simulink model "Model"  (R2020a)
settings: Solver=FixedStepAuto  StartTime=0.0  StopTime=20  RelTol=1e-3
undefined symbols (not defined in the file): A, B, Bv, Bvn, Bw, C, Cv, Cvn, Cw, d, D, DiscIntNeverNeededParam, J, K_fsfb, K_int, Kt, l, M, r, Ti, Ts
libraries: simulink x1
settings Model: Creator=User  LastModifiedBy=User
settings SolverCC: ZeroCrossControl=EnableAll  ZeroCrossAlgorithm=Adaptive
settings DebuggingCC: IgnoredZcDiagnostic=none

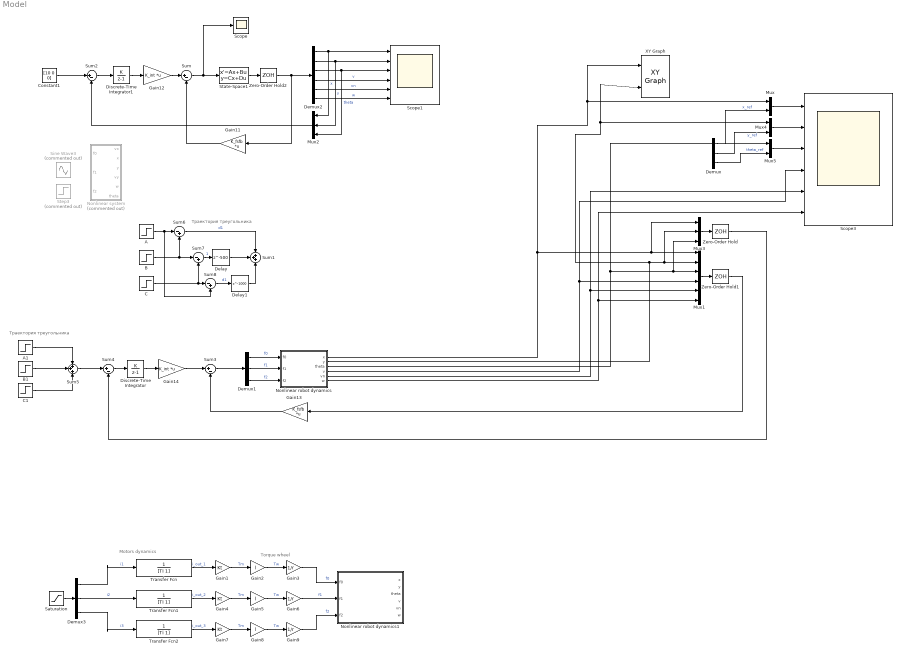
== system Model ==
  note: Motors dynamics
  note: Torque wheel
  note: Траектория треугольника
  note: Траектория треугольника
  A : Step  Time=0  Before=[0 0 0]  After=[0 0 0]  SampleTime=0
  A1 : Step  Time=0  Before=[0 0 0]  After=[0.5 -sqrt(3)/2 1]  SampleTime=0
  B : Step  Time=0  Before=[0.5 -sqrt(3)/2 0]  After=[0.5 -sqrt(3)/2 0]  SampleTime=Ts
  B1 : Step  Time=6  Before=[0 0 0]  After=[-1 0 1]  SampleTime=Ts
  C : Step  Time=0  Before=[-0.5 -sqrt(3)/2 0]  After=[-0.5 -sqrt(3)/2 0]  SampleTime=Ts
  C1 : Step  Time=12  Before=[0 0 0]  After=[0.5 sqrt(3)/2 0]  SampleTime=Ts
  Constant1 : Constant  Value=[10 0 0]
  Delay : Delay  DelayLength=500
  Delay1 : Delay  DelayLength=1000
  Demux : Demux  Outputs=3
  Demux1 : Demux  Outputs=3
  Demux2 : Demux  Outputs=6
  Demux3 : Demux  Outputs=3
  Discrete-Time Integrator : DiscreteIntegrator  IntegratorMethod=Accumulation: Forward Euler  SampleTime=Ts  ICPrevOutput=DiscIntNeverNeededParam  ICPrevScaledInput=DiscIntNeverNeededParam
  Discrete-Time Integrator1 : DiscreteIntegrator  IntegratorMethod=Accumulation: Forward Euler  SampleTime=Ts  ICPrevOutput=DiscIntNeverNeededParam  ICPrevScaledInput=DiscIntNeverNeededParam
  Gain1 : Gain  Gain=Kt
  Gain11 : Gain  Gain=K_fsfb  Multiplication=Matrix(K*u) (u vector)
  Gain12 : Gain  Gain=K_int  Multiplication=Matrix(K*u) (u vector)
  Gain13 : Gain  Gain=K_fsfb  Multiplication=Matrix(K*u) (u vector)
  Gain14 : Gain  Gain=K_int  Multiplication=Matrix(K*u) (u vector)
  Gain2 : Gain  Gain=l
  Gain3 : Gain  Gain=1/r
  Gain4 : Gain  Gain=Kt
  Gain5 : Gain  Gain=l
  Gain6 : Gain  Gain=1/r
  Gain7 : Gain  Gain=Kt
  Gain8 : Gain  Gain=l
  Gain9 : Gain  Gain=1/r
  Mux : Mux  Inputs=2
  Mux1 : Mux  Inputs=6
  Mux2 : Mux  Inputs=3
  Mux3 : Mux  Inputs=3
  Mux4 : Mux  Inputs=2
  Mux5 : Mux  Inputs=2
  Nonlinear robot dynamics : Subsystem
  Nonlinear robot dynamics1 : Subsystem
  Nonlinear system : Subsystem  Commented=on
  Saturation : Saturate  UpperLimit=4  LowerLimit=0
  Scope : Scope
  Scope1 : Scope  NumInputPorts=6
  Scope3 : Scope  NumInputPorts=6
  Sine Wave3 : Sin  Commented=on  SampleTime=0
  State-Space1 : StateSpace  A=A  B=B  C=C  D=D  InitialCondition=0  AbsoluteTolerance=-1
  Step3 : Step  Commented=on  Time=0  After=-5  SampleTime=0
  Sum{,2..4} (4 alike) : Sum  Inputs=|+-
  Sum1 : Sum  Inputs=+++
  Sum5 : Sum  Inputs=+++
  Sum6 : Sum  Inputs=|-+
  Sum7 : Sum  Inputs=|-+
  Sum8 : Sum  Inputs=|-+
  Transfer Fcn : TransferFcn  Denominator=[Ti 1]
  Transfer Fcn1 : TransferFcn  Denominator=[Ti 1]
  Transfer Fcn2 : TransferFcn  Denominator=[Ti 1]
  XY Graph : simulink/Sinks/XY Graph  xmin=-2  xmax=2  ymin=-2  ymax=2  st=-1
  Zero-Order Hold : ZeroOrderHold  SampleTime=Ts
  Zero-Order Hold1 : ZeroOrderHold  SampleTime=Ts
  Zero-Order Hold2 : ZeroOrderHold  SampleTime=Ts
  wires:
  Sum3/1 -> Demux1/1
  Demux2/1 -> Scope1/1, Mux2/1  "x"
  Demux2/2 -> Scope1/2, Mux2/2  "y"
  Demux2/3 -> Mux2/3, Scope1/3  "theta"
  Demux2/4 -> Scope1/4  "v"
  Demux2/5 -> Scope1/5  "vn"
  Demux2/6 -> Scope1/6  "w"
  State-Space1/1 -> Zero-Order Hold2/1
  Sum/1 -> Scope/1, State-Space1/1
  Gain11/1 -> Sum/2
  Constant1/1 -> Sum2/1
  Mux2/1 -> Sum2/2
  Sum2/1 -> Discrete-Time Integrator1/1
  Discrete-Time Integrator1/1 -> Gain12/1
  Gain12/1 -> Sum/1
  Discrete-Time Integrator/1 -> Gain14/1
  Sum4/1 -> Discrete-Time Integrator/1
  Gain13/1 -> Sum3/2
  Gain14/1 -> Sum3/1
  Mux3/1 -> Zero-Order Hold/1
  Mux1/1 -> Zero-Order Hold1/1
  Zero-Order Hold/1 -> Sum4/2
  Zero-Order Hold1/1 -> Gain13/1
  Zero-Order Hold2/1 -> Demux2/1, Gain11/1
  Transfer Fcn/1 -> Gain1/1  "i_out_1"
  Gain1/1 -> Gain2/1  "Tm"
  Gain2/1 -> Gain3/1  "Tw"
  Gain3/1 -> Nonlinear robot dynamics1/1(f0)  "f0"
  Mux/1 -> Scope3/1
  Mux4/1 -> Scope3/2
  Mux5/1 -> Scope3/3
  Demux/1 -> Mux/2  "x_ref"
  Demux/2 -> Mux4/2  "y_ref"
  Demux/3 -> Mux5/2  "theta_ref"
  Nonlinear robot dynamics/3(theta) -> Mux5/1, Mux3/3, Mux1/3
  Nonlinear robot dynamics/4(v) -> Scope3/4, Mux1/4
  Nonlinear robot dynamics/2(y) -> Mux4/1, XY Graph/2, Mux3/2, Mux1/2
  Nonlinear robot dynamics/1(x) -> Mux/1, XY Graph/1, Mux3/1, Mux1/1
  Nonlinear robot dynamics/5(vn) -> Scope3/5, Mux1/5
  Nonlinear robot dynamics/6(w) -> Mux1/6, Scope3/6
  Demux1/1 -> Nonlinear robot dynamics/1(f0)  "f0"
  Demux1/2 -> Nonlinear robot dynamics/2(f1)  "f1"
  Demux1/3 -> Nonlinear robot dynamics/3(f2)  "f2"
  Gain5/1 -> Gain6/1  "Tw"
  Gain4/1 -> Gain5/1  "Tm"
  Transfer Fcn1/1 -> Gain4/1  "i_out_2"
  Gain6/1 -> Nonlinear robot dynamics1/2(f1)  "f1"
  Gain7/1 -> Gain8/1  "Tm"
  Gain8/1 -> Gain9/1  "Tw"
  Gain9/1 -> Nonlinear robot dynamics1/3(f2)  "f2"
  Transfer Fcn2/1 -> Gain7/1  "i_out_3"
  Demux3/1 -> Transfer Fcn/1  "i1"
  Demux3/2 -> Transfer Fcn1/1  "i2"
  Demux3/3 -> Transfer Fcn2/1  "i3"
  Saturation/1 -> Demux3/1
  A1/1 -> Sum5/1
  A/1 -> Sum8/2, Sum6/1
  B/1 -> Sum7/1, Sum6/2
  Sum6/1 -> Sum1/1  "d1"
  C/1 -> Sum8/1, Sum7/2
  Sum7/1 -> Delay/1  "1"
  Sum8/1 -> Delay1/1  "d1"
  Delay1/1 -> Sum1/3
  Delay/1 -> Sum1/2
  B1/1 -> Sum5/2
  C1/1 -> Sum5/3
  Sum5/1 -> Sum4/1

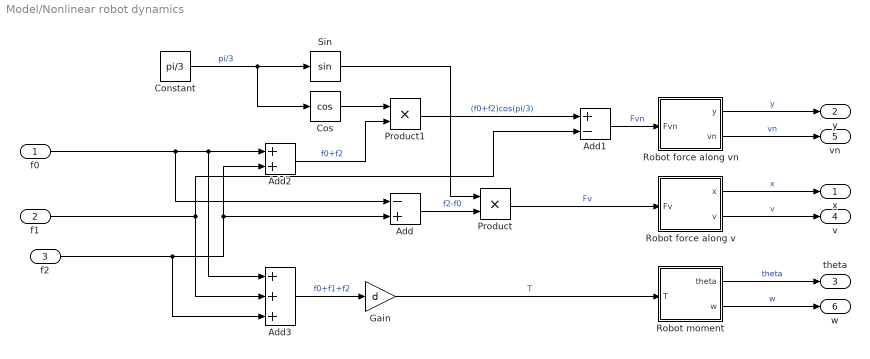
== system Model/Nonlinear robot dynamics ==
  f0 : Inport
  f1 : Inport  Port=2
  f2 : Inport  Port=3
  Add : Sum  Inputs=-+
  Add1 : Sum  Inputs=+-  AccumDataTypeStr=single  OutDataTypeStr=double
  Add2 : Sum
  Add3 : Sum  Inputs=+++
  Constant : Constant  Value=pi/3
  Cos : Trigonometry  Operator=cos
  Gain : Gain  Gain=d
  Product : Product
  Product1 : Product
  Robot force along v : Subsystem
  Robot force along vn : Subsystem
  Robot moment : Subsystem
  Sin : Trigonometry
  x : Outport
  y : Outport  Port=2
  theta : Outport  Port=3
  v : Outport  Port=4
  vn : Outport  Port=5
  w : Outport  Port=6
  wires:
  f2/1 -> Add3/3, Add2/2, Add/2
  Product1/1 -> Add1/1  "(f0+f2)cos(pi/3)"
  f0/1 -> Add/1, Add3/1, Add2/1
  Cos/1 -> Product1/1
  Product/1 -> Robot force along v/1(Fv)  "Fv"
  Sin/1 -> Product/1
  f1/1 -> Add1/2, Add3/2
  Add2/1 -> Product1/2  "f0+f2"
  Constant/1 -> Cos/1, Sin/1  "pi/3"
  Add/1 -> Product/2  "f2-f0"
  Gain/1 -> Robot moment/1(T)  "T"
  Robot force along vn/1(y) -> y/1  "y"
  Add1/1 -> Robot force along vn/1(Fvn)  "Fvn"
  Add3/1 -> Gain/1  "f0+f1+f2"
  Robot moment/1(theta) -> theta/1  "theta"
  Robot force along v/2(v) -> v/1  "v"
  Robot force along v/1(x) -> x/1  "x"
  Robot moment/2(w) -> w/1  "w"
  Robot force along vn/2(vn) -> vn/1  "vn"

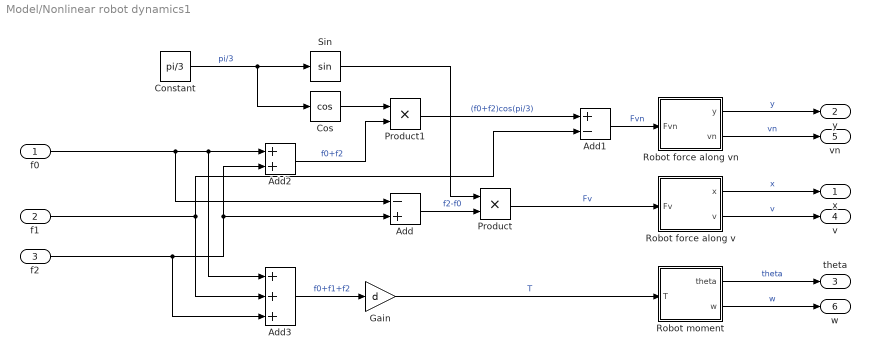
== system Model/Nonlinear robot dynamics1 ==
  f0 : Inport
  f1 : Inport  Port=2
  f2 : Inport  Port=3
  Add : Sum  Inputs=-+
  Add1 : Sum  Inputs=+-  AccumDataTypeStr=single  OutDataTypeStr=double
  Add2 : Sum
  Add3 : Sum  Inputs=+++
  Constant : Constant  Value=pi/3
  Cos : Trigonometry  Operator=cos
  Gain : Gain  Gain=d
  Product : Product
  Product1 : Product
  Robot force along v : Subsystem
  Robot force along vn : Subsystem
  Robot moment : Subsystem
  Sin : Trigonometry
  x : Outport
  y : Outport  Port=2
  theta : Outport  Port=3
  v : Outport  Port=4
  vn : Outport  Port=5
  w : Outport  Port=6
  wires:
  f2/1 -> Add3/3, Add2/2, Add/2
  Product1/1 -> Add1/1  "(f0+f2)cos(pi/3)"
  f0/1 -> Add/1, Add3/1, Add2/1
  Cos/1 -> Product1/1
  Product/1 -> Robot force along v/1(Fv)  "Fv"
  Sin/1 -> Product/1
  f1/1 -> Add1/2, Add3/2
  Add2/1 -> Product1/2  "f0+f2"
  Constant/1 -> Cos/1, Sin/1  "pi/3"
  Add/1 -> Product/2  "f2-f0"
  Gain/1 -> Robot moment/1(T)  "T"
  Robot force along vn/1(y) -> y/1  "y"
  Add1/1 -> Robot force along vn/1(Fvn)  "Fvn"
  Add3/1 -> Gain/1  "f0+f1+f2"
  Robot moment/1(theta) -> theta/1  "theta"
  Robot force along v/2(v) -> v/1  "v"
  Robot force along v/1(x) -> x/1  "x"
  Robot moment/2(w) -> w/1  "w"
  Robot force along vn/2(vn) -> vn/1  "vn"

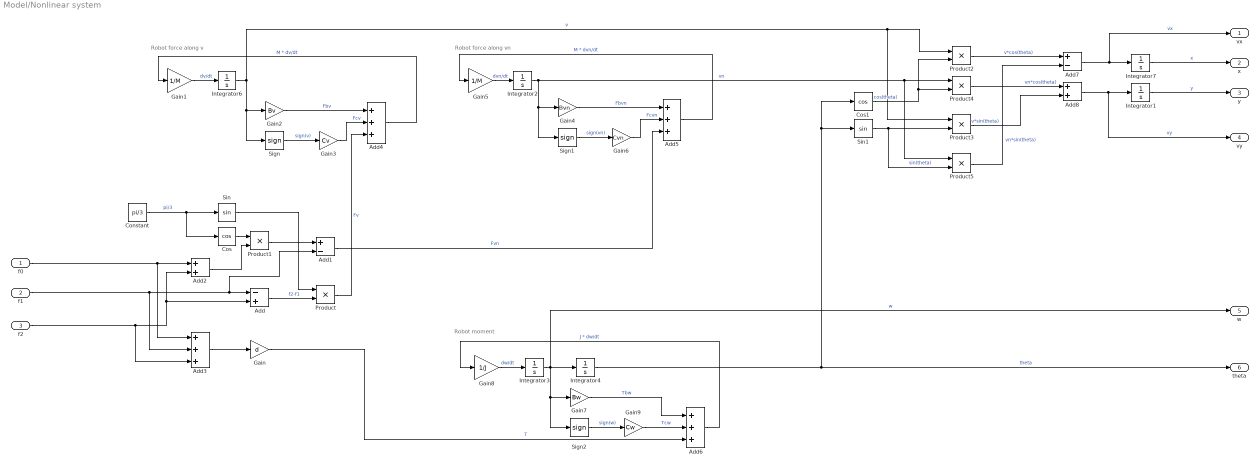
== system Model/Nonlinear system ==
  note: Robot force along vn
  note: Robot force along v
  note: Robot moment
  f0 : Inport
  f1 : Inport  Port=2
  f2 : Inport  Port=3
  Add : Sum  Inputs=-+
  Add1 : Sum  Inputs=+-
  Add2 : Sum
  Add{3..6} (4 alike) : Sum  Inputs=+++
  Add7 : Sum  Inputs=+-
  Add8 : Sum
  Constant : Constant  Value=pi/3
  Cos : Trigonometry  Operator=cos
  Cos1 : Trigonometry  Operator=cos
  Gain : Gain  Gain=d
  Gain1 : Gain  Gain=1/M
  Gain2 : Gain  Gain=Bv
  Gain3 : Gain  Gain=Cv
  Gain4 : Gain  Gain=Bvn
  Gain5 : Gain  Gain=1/M
  Gain6 : Gain  Gain=Cvn
  Gain7 : Gain  Gain=Bw
  Gain8 : Gain  Gain=1/J
  Gain9 : Gain  Gain=Cw
  Integrator1 : Integrator  ContinuousStateAttributes='y'
  Integrator2 : Integrator  ContinuousStateAttributes='vn'
  Integrator3 : Integrator  ContinuousStateAttributes='w'
  Integrator4 : Integrator  ContinuousStateAttributes='theta'
  Integrator6 : Integrator  ContinuousStateAttributes='v'
  Integrator7 : Integrator  ContinuousStateAttributes='x'
  Product{,1..5} (6 alike) : Product
  Sign : Signum
  Sign1 : Signum
  Sign2 : Signum
  Sin : Trigonometry
  Sin1 : Trigonometry
  vx : Outport
  x : Outport  Port=2
  y : Outport  Port=3
  vy : Outport  Port=4
  w : Outport  Port=5
  theta : Outport  Port=6
  wires:
  Gain6/1 -> Add5/2  "Fcvn"
  Sin1/1 -> Product5/2, Product3/2  "sin(theta)"
  f1/1 -> Add3/2, Add1/2, Add/1
  Constant/1 -> Cos/1, Sin/1  "pi/3"
  Product4/1 -> Add8/1  "vn*cos(theta)"
  Integrator4/1 -> Cos1/1, Sin1/1, theta/1  "theta"
  f0/1 -> Add3/1, Add2/1
  Sign2/1 -> Gain9/1  "sign(w)"
  Product/1 -> Add4/3  "Fv"
  f2/1 -> Add3/3, Add2/2, Add/2
  Add6/1 -> Gain8/1  "J * dw/dt"
  Integrator2/1 -> Sign1/1, Gain4/1, Product5/1, Product4/1  "vn"
  Gain7/1 -> Add6/1  "Tbw"
  Product5/1 -> Add7/2  "vn*sin(theta)"
  Gain9/1 -> Add6/2  "Tcw"
  Cos1/1 -> Product4/2, Product2/2  "cos(theta)"
  Add2/1 -> Product1/2
  Integrator6/1 -> Product3/1, Product2/1, Sign/1, Gain2/1  "v"
  Cos/1 -> Product1/1
  Gain5/1 -> Integrator2/1  "dvn/dt"
  Gain4/1 -> Add5/1  "Fbvn"
  Integrator1/1 -> y/1  "y"
  Add8/1 -> vy/1, Integrator1/1  "vy"
  Add3/1 -> Gain/1
  Add4/1 -> Gain1/1  "M * dv/dt"
  Add1/1 -> Add5/3  "Fvn"
  Product1/1 -> Add1/1
  Add/1 -> Product/2  "f2-f1"
  Gain/1 -> Add6/3  "T"
  Sin/1 -> Product/1
  Gain1/1 -> Integrator6/1  "dv/dt"
  Gain3/1 -> Add4/2  "Fcv"
  Add5/1 -> Gain5/1  "M * dvn/dt"
  Sign/1 -> Gain3/1  "sign(v)"
  Gain2/1 -> Add4/1  "Fbv"
  Product2/1 -> Add7/1  "v*cos(theta)"
  Sign1/1 -> Gain6/1  "sign(vn)"
  Add7/1 -> vx/1, Integrator7/1  "vx"
  Integrator3/1 -> w/1, Integrator4/1, Sign2/1, Gain7/1  "w"
  Product3/1 -> Add8/2  "v*sin(theta)"
  Gain8/1 -> Integrator3/1  "dw/dt"
  Integrator7/1 -> x/1  "x"

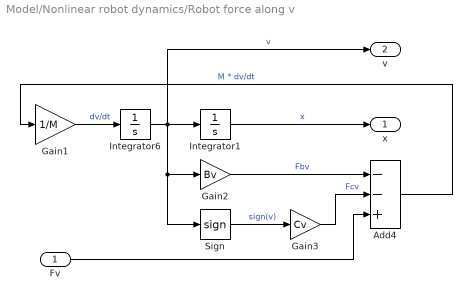
== system Model/Nonlinear robot dynamics/Robot force along v ==
  Fv : Inport
  Add4 : Sum  Inputs=--+
  Gain1 : Gain  Gain=1/M
  Gain2 : Gain  Gain=Bv
  Gain3 : Gain  Gain=Cv
  Integrator1 : Integrator  ContinuousStateAttributes='x'
  Integrator6 : Integrator  ContinuousStateAttributes='v'
  Sign : Signum
  x : Outport
  v : Outport  Port=2
  wires:
  Fv/1 -> Add4/3
  Sign/1 -> Gain3/1  "sign(v)"
  Gain2/1 -> Add4/1  "Fbv"
  Gain3/1 -> Add4/2  "Fcv"
  Integrator1/1 -> x/1  "x"
  Integrator6/1 -> v/1, Integrator1/1, Sign/1, Gain2/1  "v"
  Gain1/1 -> Integrator6/1  "dv/dt"
  Add4/1 -> Gain1/1  "M * dv/dt"

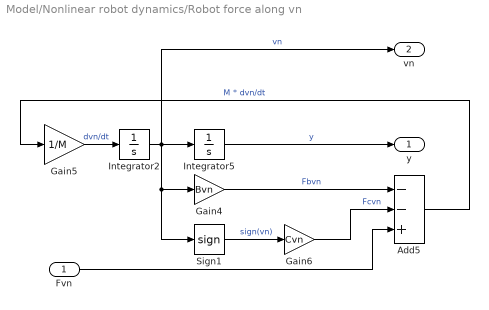
== system Model/Nonlinear robot dynamics/Robot force along vn ==
  Fvn : Inport
  Add5 : Sum  Inputs=--+
  Gain4 : Gain  Gain=Bvn
  Gain5 : Gain  Gain=1/M
  Gain6 : Gain  Gain=Cvn
  Integrator2 : Integrator  ContinuousStateAttributes='vn'
  Integrator5 : Integrator  ContinuousStateAttributes='y'
  Sign1 : Signum
  y : Outport
  vn : Outport  Port=2
  wires:
  Gain5/1 -> Integrator2/1  "dvn/dt"
  Integrator2/1 -> vn/1, Integrator5/1, Sign1/1, Gain4/1  "vn"
  Gain6/1 -> Add5/2  "Fcvn"
  Fvn/1 -> Add5/3
  Add5/1 -> Gain5/1  "M * dvn/dt"
  Sign1/1 -> Gain6/1  "sign(vn)"
  Gain4/1 -> Add5/1  "Fbvn"
  Integrator5/1 -> y/1  "y"

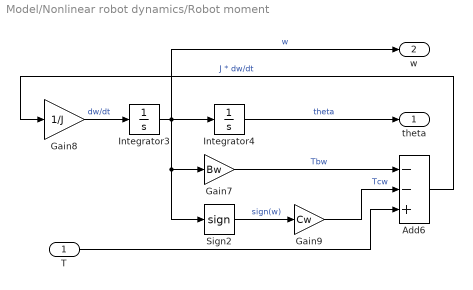
== system Model/Nonlinear robot dynamics/Robot moment ==
  T : Inport
  Add6 : Sum  Inputs=--+
  Gain7 : Gain  Gain=Bw
  Gain8 : Gain  Gain=1/J
  Gain9 : Gain  Gain=Cw
  Integrator3 : Integrator  ContinuousStateAttributes='w'
  Integrator4 : Integrator  ContinuousStateAttributes='theta'
  Sign2 : Signum
  theta : Outport
  w : Outport  Port=2
  wires:
  Integrator3/1 -> w/1, Integrator4/1, Sign2/1, Gain7/1  "w"
  Gain8/1 -> Integrator3/1  "dw/dt"
  Add6/1 -> Gain8/1  "J * dw/dt"
  Gain9/1 -> Add6/2  "Tcw"
  Gain7/1 -> Add6/1  "Tbw"
  Sign2/1 -> Gain9/1  "sign(w)"
  Integrator4/1 -> theta/1  "theta"
  T/1 -> Add6/3

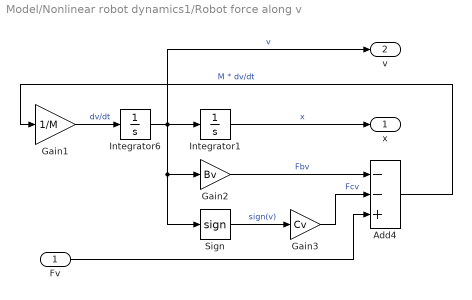
== system Model/Nonlinear robot dynamics1/Robot force along v ==
  Fv : Inport
  Add4 : Sum  Inputs=--+
  Gain1 : Gain  Gain=1/M
  Gain2 : Gain  Gain=Bv
  Gain3 : Gain  Gain=Cv
  Integrator1 : Integrator  ContinuousStateAttributes='x'
  Integrator6 : Integrator  ContinuousStateAttributes='v'
  Sign : Signum
  x : Outport
  v : Outport  Port=2
  wires:
  Fv/1 -> Add4/3
  Sign/1 -> Gain3/1  "sign(v)"
  Gain2/1 -> Add4/1  "Fbv"
  Gain3/1 -> Add4/2  "Fcv"
  Integrator1/1 -> x/1  "x"
  Integrator6/1 -> v/1, Integrator1/1, Sign/1, Gain2/1  "v"
  Gain1/1 -> Integrator6/1  "dv/dt"
  Add4/1 -> Gain1/1  "M * dv/dt"

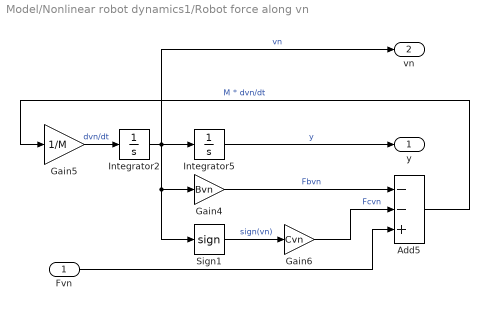
== system Model/Nonlinear robot dynamics1/Robot force along vn ==
  Fvn : Inport
  Add5 : Sum  Inputs=--+
  Gain4 : Gain  Gain=Bvn
  Gain5 : Gain  Gain=1/M
  Gain6 : Gain  Gain=Cvn
  Integrator2 : Integrator  ContinuousStateAttributes='vn'
  Integrator5 : Integrator  ContinuousStateAttributes='y'
  Sign1 : Signum
  y : Outport
  vn : Outport  Port=2
  wires:
  Gain5/1 -> Integrator2/1  "dvn/dt"
  Integrator2/1 -> vn/1, Integrator5/1, Sign1/1, Gain4/1  "vn"
  Gain6/1 -> Add5/2  "Fcvn"
  Fvn/1 -> Add5/3
  Add5/1 -> Gain5/1  "M * dvn/dt"
  Sign1/1 -> Gain6/1  "sign(vn)"
  Gain4/1 -> Add5/1  "Fbvn"
  Integrator5/1 -> y/1  "y"

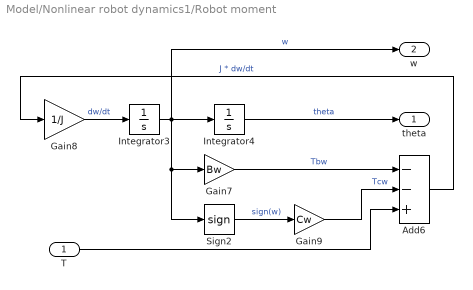
== system Model/Nonlinear robot dynamics1/Robot moment ==
  T : Inport
  Add6 : Sum  Inputs=--+
  Gain7 : Gain  Gain=Bw
  Gain8 : Gain  Gain=1/J
  Gain9 : Gain  Gain=Cw
  Integrator3 : Integrator  ContinuousStateAttributes='w'
  Integrator4 : Integrator  ContinuousStateAttributes='theta'
  Sign2 : Signum
  theta : Outport
  w : Outport  Port=2
  wires:
  Integrator3/1 -> w/1, Integrator4/1, Sign2/1, Gain7/1  "w"
  Gain8/1 -> Integrator3/1  "dw/dt"
  Add6/1 -> Gain8/1  "J * dw/dt"
  Gain9/1 -> Add6/2  "Tcw"
  Gain7/1 -> Add6/1  "Tbw"
  Sign2/1 -> Gain9/1  "sign(w)"
  Integrator4/1 -> theta/1  "theta"
  T/1 -> Add6/3
